simulink model "task2"  (R2022a)
settings: Solver=VariableStepAuto  StartTime=0.0  StopTime=2  RelTol=1e-3
settings Model: Creator=novik  LastModifiedBy=novik

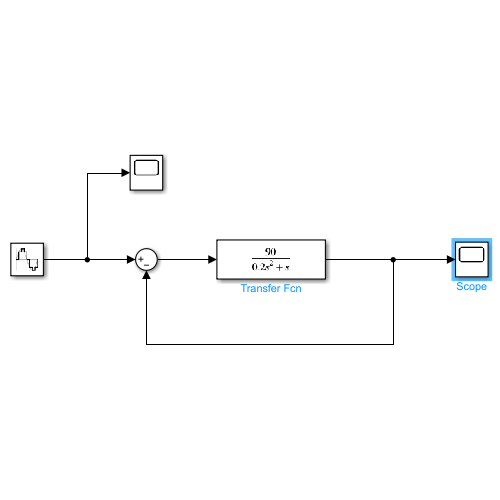
[thumbnail: Simulink's stored preview of the top-level diagram]
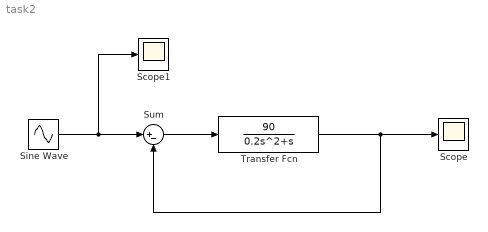
== system task2 ==
  Scope : Scope
  Scope1 : Scope
  Sine Wave : Sin  Amplitude=100  Frequency=500  SampleTime=0.0001
  Sum : Sum  Inputs=|+-
  Transfer Fcn : TransferFcn  Numerator=[90]  Denominator=[0.2 1 0]
  wires:
  Sine Wave/1 -> Scope1/1, Sum/1
  Sum/1 -> Transfer Fcn/1
  Transfer Fcn/1 -> Sum/2, Scope/1
